simulink model "Pedestrian_CarCamera"  (R2024b)
settings: Solver=VariableStepAuto  StartTime=0.0  StopTime=inf  RelTol=1e-3
values from neighbouring files (symbols this model uses):
  C = [1 0 0 0; 0 1 0 0]    [Car_test_UDP.m]    (also in Final_Code_GPS.m; Final_Code_plotting_reset_kalman.m; KalmanFilter.m)
libraries: sim3dautolib x2, sim3dlib x1
settings Model: Creator=The MathWorks, Inc.  LastModifiedBy=ritvi
settings SolverCC: AlgebraicLoopSolver=TrustRegion
settings OptimizationCC: ReuseModelBlockBuffer=off
settings DebuggingCC: UnconnectedInputMsg=warning  UnconnectedOutputMsg=warning  UnconnectedLineMsg=warning  SymbolicDimsDataTypeCodeGenerationDiagnostic=none
settings ModelReferenceCC: EnableRefExpFcnMdlSchedulingChecks=on
settings RTWCC: GPUComputeCapability=3.5  DLArmComputeVersion=19.05

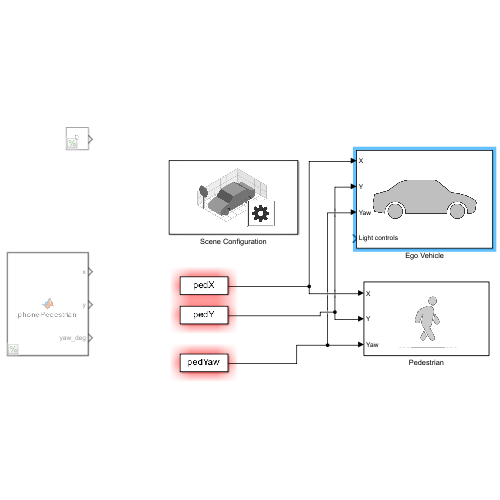
[thumbnail: Simulink's stored preview of the top-level diagram]
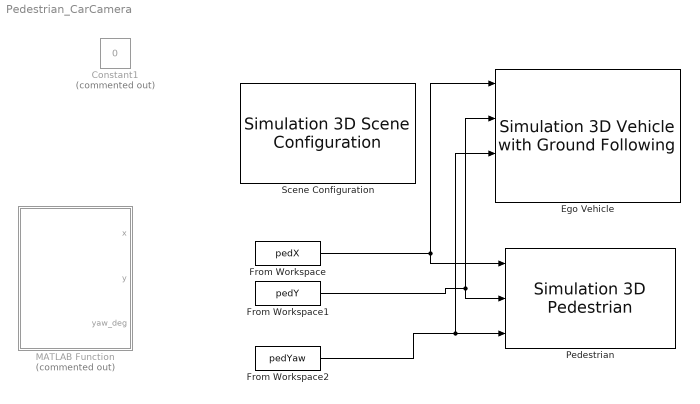
== system Pedestrian_CarCamera ==
  Constant1 : Constant  Commented=on  Value=0
  Ego Vehicle : sim3dautolib/Simulation 3D Vehicle with Ground Following  Priority=-1  PassVehMesh=Box truck  MeshPath=/MathWorksSimulation/Vehicles/Muscle/Meshes/SK_MuscleCar.SK_MuscleCar  TrackWidth=1.9  WheelBase=3  WheelRadius=0.35  VehColor=Red  InitialPos=[10, 10, 0]  InitialRot=[0, 0, 90]  ActorName=SimulinkVehicle1  SampleTime=-1  ActorType=SimulinkVehicle  ID=1  aMode=3  ActorTag=SimulinkVehicle1  CoordinateScheme=ISO  VehLightsControl=on  HeadlightColor=[ 1, 1, 1 ]  HighBeamIntensity=100000  LowBeamIntensity=60000  HighBeamConeAngle=70  LowBeamConeAngle=70  LeftHeadlightOrientation=[ 0, 0 ]  RightHeadlightOrientation=[ 0, 0 ]  BrakelightIntensity=500  ReverselightIntensity=500  SignallightIntensity=500  SignallightPeriod=1  SignalPulseWidth=50  TransformOutportEnabled=off
      settings: LibrarySourceBlock=drivingsim3d/Simulation 3D Vehicle with Ground Following
  From Workspace : FromWorkspace  VariableName=pedX
  From Workspace1 : FromWorkspace  VariableName=pedY
  From Workspace2 : FromWorkspace  VariableName=pedYaw
  MATLAB Function : MATLAB Function  Commented=on  TreatAsAtomicUnit=on
  Pedestrian : sim3dautolib/Simulation 3D Pedestrian  Priority=-1  PedestrianType=Female 1  Scale=[1, 1, 1]  InitialPos=[10, 10, 0]  InitialYaw=0  ActorName=SimulinkPedestrian1  SampleTime=-1  ActorType=SimulinkPedestrian  ActorTag=SimulinkPedestrian1  ID=1  aMode=3  CoordinateScheme=ISO  TransformOutportEnabled=off
      settings: LibrarySourceBlock=drivingsim3d/Simulation 3D Pedestrian
  Scene Configuration : sim3dlib/Simulation 3D Scene Configuration  Priority=0  ProjectFormat=Unreal Editor  SceneDesc=Large parking lot  ProjectName=C:\Program Files\MATLAB\R2024b\toolbox\shared\sim3d_projects\automotive_project_windows\UE\WindowsNoEditor\VehicleSimulation.exe  ScenePath=/Game/Maps/HwStrght  UEProjPath=C:\Local\AutoVrtlEnv\AutoVrtlEnv.uproject  EnableOpenDRIVE=off  vehTagList={'Custom';'Scene Origin';'SimulinkVehicle1'}  vehTag=SimulinkVehicle1  FreeCameraInitialTranslation=[0, 0,10]  FreeCameraDefaultInitialTranslation=[-6, 0, 2]  FreeCameraInitialRotation=[0, 0, 0]  FreeCameraDefaultInitialRotation=[0, -15, 0]  OpVisEn=off  Ts=1/60  EnableWindow=on  EnableRemoteAccess=off  EnableWeather=off  SunAzimuth=183.600  SunAltitude=0.0  EnableGeospatialSun=off  Latitude=0  Longitude=0  Date=2023-01-01  Time=10:30:00  GeoTimeZone=-5.0  SunDaylightSaving=off  wind=1  clouds=50.0  EnableVolumetricClouds=off  CloudCoverage=0  CloudAltitude=6  fog=0.0  rain=18.0  RaindropsEffect=off  SnowDensity=0  EnableGeospatial=off  UseTrueOrigin=off  OriginHeight=200  OriginLatitude=40.744652  OriginLongitude=-73.988864  MapStyle=Aerial  AdditionalAssetIDs=[]  UseAdvancedSunSky=off  SolarTime=11  TimeZone=-5  Day=21  Month=9  Year=2022  UseDaylightSavingTime=on  DSTStartDay=10  DSTStartMonth=3  DSTEndDay=3  DSTEndMonth=11  DSTSwitchHour=2  sensorTag=MainCamera2  sensorId=2  sensorName=MainCamera2  mountLoc=Origin  offsetFlag=off  tmountOffset=[0, 0, 0]  rmountOffset=[0, 0, 0]  HorizontalResolution=1280  VerticalResolution=720  HorizontalFOV=60  mountPoint=[0 0 0]  mountOrientation=[0 0 0]  aMode=3  ID=2  GeoTrigger=Inactive
      settings: LibrarySourceBlock=drivingsim3d/Simulation 3D Scene Configuration
  wires:
  From Workspace/1 -> Pedestrian/1, Ego Vehicle/1
  From Workspace1/1 -> Ego Vehicle/2, Pedestrian/2
  From Workspace2/1 -> Ego Vehicle/3, Pedestrian/3

== matlab function Pedestrian_CarCamera/MATLAB Function ==
  data: x output; y output; yaw_deg output
function [x, y, yaw_deg] = phonePedestrian()
%#codegen

% Read MATLAB workspace value
coder.extrinsic('evalin');

% -------------------------------------------------
% PARAMETERS (tune if needed)
% -------------------------------------------------
v  = 1.2;        % walking speed (m/s)
Ts = 0.02;       % simulation step (s)

% -------------------------------------------------
% STATE (persistent)
% -------------------------------------------------
persistent yaw x_pos y_pos
if isempty(yaw)
    yaw   = 0.0;   % radians
    x_pos = 0.0;   % meters
    y_pos = 0.0;   % meters
end

% -------------------------------------------------
% INPUT: phone gyro (rad/s)
% -------------------------------------------------
wz = 0.0;
wz = evalin('base','YawRate');

% -------------------------------------------------
% UPDATE STATE
% -------------------------------------------------
yaw = yaw + wz * Ts;

x_pos = x_pos + v * cos(yaw) * Ts+ 10;
y_pos = y_pos + v * sin(yaw) * Ts + 10;

% -------------------------------------------------
% OUTPUTS
% -------------------------------------------------
x = x_pos;
y = y_pos;
yaw_deg = yaw * 180/pi;   % Pedestrian expects degrees
